simulink model "thermal_analysis"  (R2023b)
settings: Solver=VariableStepAuto  StartTime=0.0  StopTime=1  RelTol=1e-3
values from neighbouring files (symbols this model uses):
  air_temp_init = 75    [run_thermal_analysis.m]
  cap_loss = 194.3    [run_thermal_analysis.m]
  case_temp_init = 75    [run_thermal_analysis.m]
  EMI_loss = 147.1    [run_thermal_analysis.m]
  jyouge_loss = 51.3    [run_thermal_analysis.m]
  module_loss = 426.1    [run_thermal_analysis.m]
  OutTanshi_loss = 94.5    [run_thermal_analysis.m]
  PDC_loss = 16.7    [run_thermal_analysis.m]
  PN_loss = 22.3    [run_thermal_analysis.m]
  PN_temp_init = 82    [run_thermal_analysis.m]
  tanshidai_loss = 514.1    [run_thermal_analysis.m]
libraries: spsSeriesRLCBranchLib x29, spsGroundLib x19, spsControlledCurrentSourceLib x8, spsVoltageMeasurementLib x8, spsACCurrentSourceLib x7, spsDCVoltageSourceLib x3, spsCurrentMeasurementLib x1, sps_lib x1
settings Model: Creator=snow_  LastModifiedBy=snow_
settings DataIOCC: ReturnWorkspaceOutputs=off

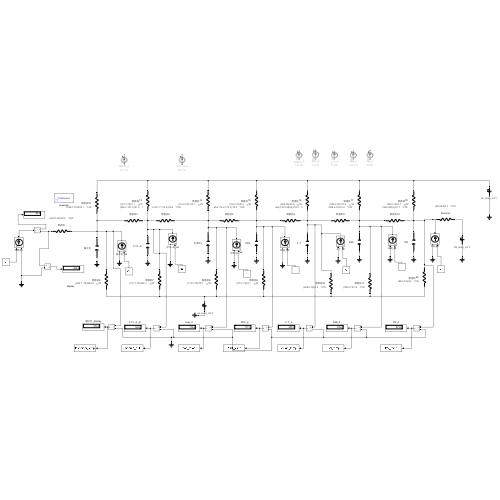
[thumbnail: Simulink's stored preview of the top-level diagram]
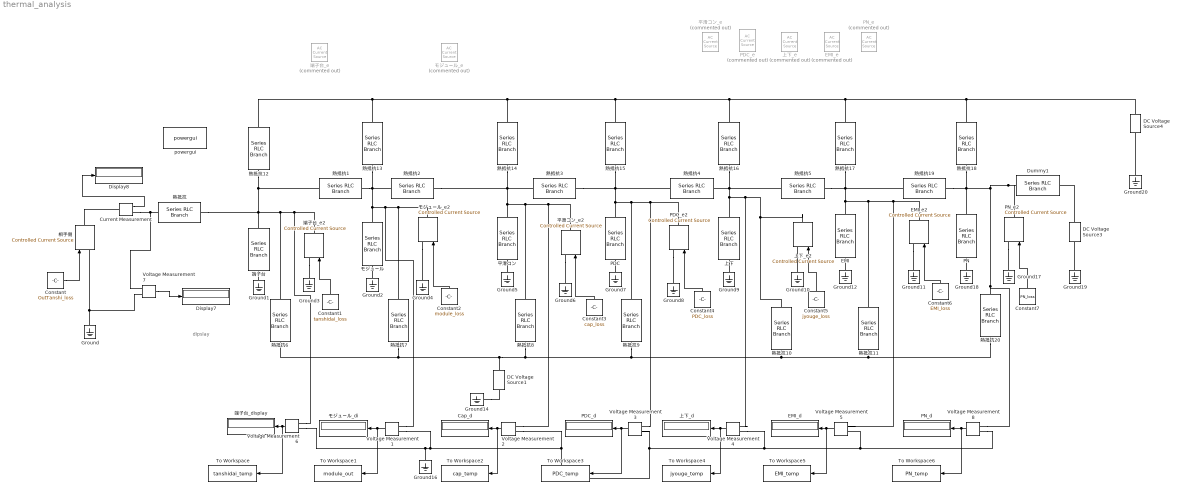
== system thermal_analysis ==
  note: dipslay
  Cap_d : Display
  Constant : Constant  Value=OutTanshi_loss
  Constant1 : Constant  Value=tanshidai_loss
  Constant2 : Constant  Value=module_loss
  Constant3 : Constant  Value=cap_loss
  Constant4 : Constant  Value=PDC_loss
  Constant5 : Constant  Value=jyouge_loss
  Constant6 : Constant  Value=EMI_loss
  Constant7 : Constant  Value=PN_loss
  Current Measurement : spsCurrentMeasurementLib/Current Measurement  PhasorSimulation=off  OutputType=Complex  PSBequivalent=0
  DC Voltage Source1 : spsDCVoltageSourceLib/DC Voltage Source  Amplitude=case_temp_init  Measurements=None
      settings: AttributesFormatString=%<Amplitude>℃
  DC Voltage Source3 : spsDCVoltageSourceLib/DC Voltage Source  Amplitude=PN_temp_init  Measurements=None
      settings: AttributesFormatString=%<Amplitude>℃
  DC Voltage Source4 : spsDCVoltageSourceLib/DC Voltage Source  Amplitude=air_temp_init  Measurements=None
      settings: AttributesFormatString=%<Amplitude>℃
  Display7 : Display
  Display8 : Display
  Dummy1 : spsSeriesRLCBranchLib/Series RLC Branch  LConnTagsString=__new0  RConnTagsString=__new0  BranchType=R  Resistance=(88-82)/50.7  Inductance=1e-3  SetiL0=off  InitialCurrent=0  Capacitance=0.1  Setx0=off  InitialVoltage=0  Measurements=None
      settings: AttributesFormatString=%<Resistance>　℃/W
  EMI : spsSeriesRLCBranchLib/Series RLC Branch  LConnTagsString=__new0  RConnTagsString=__new0  BranchType=C  Resistance=1  Inductance=1e-3  SetiL0=off  InitialCurrent=0  Capacitance=0.1  Setx0=off  InitialVoltage=0  Measurements=None
  EMI_d : Display
  EMI_e : spsACCurrentSourceLib/AC Current Source  Commented=on  Amplitude=147.1  Phase=0  Frequency=0  SampleTime=0  Measurements=None
      settings: AttributesFormatString=%<Amplitude>W  LibrarySourceBlock=sps_lib/Sources/AC Current Source
  EMI_e2 : spsControlledCurrentSourceLib/Controlled Current Source  Initialize=on  Source_Type=AC  Amplitude=0  Phase=0  Frequency=0  Measurements=None
  Ground{,1..12,14,16..20} (19 alike) : spsGroundLib/Ground  LConnTagsString=a
  PDC : spsSeriesRLCBranchLib/Series RLC Branch  LConnTagsString=__new0  RConnTagsString=__new0  BranchType=C  Resistance=1  Inductance=1e-3  SetiL0=off  InitialCurrent=0  Capacitance=0.1  Setx0=off  InitialVoltage=0  Measurements=None
  PDC_d : Display
  PDC_e : spsACCurrentSourceLib/AC Current Source  Commented=on  Amplitude=16.7  Phase=0  Frequency=0  SampleTime=0  Measurements=None
      settings: AttributesFormatString=%<Amplitude>W  LibrarySourceBlock=sps_lib/Sources/AC Current Source
  PDC_e2 : spsControlledCurrentSourceLib/Controlled Current Source  Initialize=on  Source_Type=AC  Amplitude=0  Phase=0  Frequency=0  Measurements=None
  PN : spsSeriesRLCBranchLib/Series RLC Branch  LConnTagsString=__new0  RConnTagsString=__new0  BranchType=C  Resistance=1  Inductance=1e-3  SetiL0=off  InitialCurrent=0  Capacitance=0.1  Setx0=off  InitialVoltage=0  Measurements=None
  PN_d : Display
  PN_e : spsACCurrentSourceLib/AC Current Source  Commented=on  Amplitude=22.3  Phase=0  Frequency=0  SampleTime=0  Measurements=None
      settings: AttributesFormatString=%<Amplitude>W  LibrarySourceBlock=sps_lib/Sources/AC Current Source
  PN_e2 : spsControlledCurrentSourceLib/Controlled Current Source  Initialize=on  Source_Type=AC  Amplitude=0  Phase=0  Frequency=0  Measurements=None
  To Workspace : ToWorkspace  VariableName=tanshidai_temp  SampleTime=-1
  To Workspace1 : ToWorkspace  VariableName=module_out  SampleTime=-1
  To Workspace2 : ToWorkspace  VariableName=cap_temp  SampleTime=-1
  To Workspace3 : ToWorkspace  VariableName=PDC_temp  SampleTime=-1
  To Workspace4 : ToWorkspace  VariableName=jyouge_temp  SampleTime=-1
  To Workspace5 : ToWorkspace  VariableName=EMI_temp  SampleTime=-1
  To Workspace6 : ToWorkspace  VariableName=PN_temp  SampleTime=-1
  Voltage Measurement{1..8} (8 alike) : spsVoltageMeasurementLib/Voltage Measurement  PhasorSimulation=off  OutputType=Complex  PSBequivalent=0
  powergui : sps_lib/powergui  Priority=1  SimulationMode=Continuous  SampleTime=50e-6  frequency=60  Iterations=50  frequencyindice=0  Pbase=100e6  ErrMax=1e-4  UnitsV=kV  UnitsW=MW  buscounter=0  FunctionMessages=off  echomessages=off  EnableUseOfTLC=off  CurrentSourceSwitches=off  DisableSnubberDevices=off  DisableRonSwitches=off  DisableVfSwitches=off  DisplayEquations=off  AutomaticDiscreteSolvers=off  SolverType=Tustin/Backward Euler (TBE)  Interpol=off  ExternalGateDelay=off  methode=off  Ts=100  x0status=blocks  SPID=on  SwTol=0  HookPort=off  NonlinearTolerance=1e-4  nMaxIteration=100  ContinueOnMaxIteration=off  RestoreLinks=warning  ResistiveCurrentMeasurement=off  Frange=[0:2:500]  Ylog=off  Xlog=on  ShowGrid=off  save=off  variable=ZData  structure=0  ZoomFFT=off  StartTime=0.0  cycles=1  DisplayStyle=1  fundamental=60  FreqAxis=off  MaxFrequency=1000  frequencyindicesteady=1  RmsSteady=1  display=off
  モジュール : spsSeriesRLCBranchLib/Series RLC Branch  LConnTagsString=__new0  RConnTagsString=__new0  BranchType=C  Resistance=1  Inductance=1e-3  SetiL0=off  InitialCurrent=0  Capacitance=0.1  Setx0=off  InitialVoltage=0  Measurements=None
  モジュール_di : Display
  モジュール_e : spsACCurrentSourceLib/AC Current Source  Commented=on  Amplitude=426.1  Phase=0  Frequency=0  SampleTime=0  Measurements=None
      settings: AttributesFormatString=%<Amplitude>W  LibrarySourceBlock=sps_lib/Sources/AC Current Source
  モジュール_e2 : spsControlledCurrentSourceLib/Controlled Current Source  Initialize=on  Source_Type=AC  Amplitude=0  Phase=0  Frequency=0  Measurements=None
  上下 : spsSeriesRLCBranchLib/Series RLC Branch  LConnTagsString=__new0  RConnTagsString=__new0  BranchType=C  Resistance=1  Inductance=1e-3  SetiL0=off  InitialCurrent=0  Capacitance=0.1  Setx0=off  InitialVoltage=0  Measurements=None
  上下_d : Display
  上下_e : spsACCurrentSourceLib/AC Current Source  Commented=on  Amplitude=51.3  Phase=0  Frequency=0  SampleTime=0  Measurements=None
      settings: AttributesFormatString=%<Amplitude>W  LibrarySourceBlock=sps_lib/Sources/AC Current Source
  上下_e2 : spsControlledCurrentSourceLib/Controlled Current Source  Initialize=on  Source_Type=AC  Amplitude=0  Phase=0  Frequency=0  Measurements=None
  平滑コン : spsSeriesRLCBranchLib/Series RLC Branch  LConnTagsString=__new0  RConnTagsString=__new0  BranchType=C  Resistance=1  Inductance=1e-3  SetiL0=off  InitialCurrent=0  Capacitance=0.1  Setx0=off  InitialVoltage=0  Measurements=None
  平滑コン_e : spsACCurrentSourceLib/AC Current Source  Commented=on  Amplitude=194.3  Phase=0  Frequency=0  SampleTime=0  Measurements=None
      settings: AttributesFormatString=%<Amplitude>W  LibrarySourceBlock=sps_lib/Sources/AC Current Source
  平滑コン_e2 : spsControlledCurrentSourceLib/Controlled Current Source  Initialize=on  Source_Type=AC  Amplitude=0  Phase=0  Frequency=0  Measurements=None
  熱抵抗 : spsSeriesRLCBranchLib/Series RLC Branch  LConnTagsString=__new0  RConnTagsString=__new0  BranchType=R  Resistance=(269.7-82)/94.5  Inductance=1e-3  SetiL0=off  InitialCurrent=0  Capacitance=0.1  Setx0=off  InitialVoltage=0  Measurements=None
      settings: AttributesFormatString=%<Resistance>　℃/W
  熱抵抗1 : spsSeriesRLCBranchLib/Series RLC Branch  LConnTagsString=__new0  RConnTagsString=__new0  BranchType=R  Resistance=(269.7-101.7)/51.5  Inductance=1e-3  SetiL0=off  InitialCurrent=0  Capacitance=0.1  Setx0=off  InitialVoltage=0  Measurements=None
      settings: AttributesFormatString=%<Resistance>　℃/W
  熱抵抗10 : spsSeriesRLCBranchLib/Series RLC Branch  LConnTagsString=__new0  RConnTagsString=__new0  BranchType=R  Resistance=(289.6-75)/3.5  Inductance=1e-3  SetiL0=off  InitialCurrent=0  Capacitance=0.1  Setx0=off  InitialVoltage=0  Measurements=None
      settings: AttributesFormatString=%<Resistance>　℃/W
  熱抵抗11 : spsSeriesRLCBranchLib/Series RLC Branch  LConnTagsString=__new0  RConnTagsString=__new0  BranchType=R  Resistance=(198.2-75)/12  Inductance=1e-3  SetiL0=off  InitialCurrent=0  Capacitance=0.1  Setx0=off  InitialVoltage=0  Measurements=None
      settings: AttributesFormatString=%<Resistance>　℃/W
  熱抵抗12 : spsSeriesRLCBranchLib/Series RLC Branch  LConnTagsString=__new0  RConnTagsString=__new0  BranchType=R  Resistance=(269.7-75)/260.1  Inductance=1e-3  SetiL0=off  InitialCurrent=0  Capacitance=0.1  Setx0=off  InitialVoltage=0  Measurements=None
      settings: AttributesFormatString=%<Resistance>　℃/W
  熱抵抗13 : spsSeriesRLCBranchLib/Series RLC Branch  LConnTagsString=__new0  RConnTagsString=__new0  BranchType=R  Resistance=(101.7-75)/1.1  Inductance=1e-3  SetiL0=off  InitialCurrent=0  Capacitance=0.1  Setx0=off  InitialVoltage=0  Measurements=None
      settings: AttributesFormatString=%<Resistance>　℃/W
  熱抵抗14 : spsSeriesRLCBranchLib/Series RLC Branch  LConnTagsString=__new0  RConnTagsString=__new0  BranchType=R  Resistance=(174.2-75)/112.1  Inductance=1e-3  SetiL0=off  InitialCurrent=0  Capacitance=0.1  Setx0=off  InitialVoltage=0  Measurements=None
      settings: AttributesFormatString=%<Resistance>　℃/W
  熱抵抗15 : spsSeriesRLCBranchLib/Series RLC Branch  LConnTagsString=__new0  RConnTagsString=__new0  BranchType=R  Resistance=(176.7-75)/8.4  Inductance=1e-3  SetiL0=off  InitialCurrent=0  Capacitance=0.1  Setx0=off  InitialVoltage=0  Measurements=None
      settings: AttributesFormatString=%<Resistance>　℃/W
  熱抵抗16 : spsSeriesRLCBranchLib/Series RLC Branch  LConnTagsString=__new0  RConnTagsString=__new0  BranchType=R  Resistance=(289-75)/20.9  Inductance=1e-3  SetiL0=off  InitialCurrent=0  Capacitance=0.1  Setx0=off  InitialVoltage=0  Measurements=None
      settings: AttributesFormatString=%<Resistance>　℃/W
  熱抵抗17 : spsSeriesRLCBranchLib/Series RLC Branch  LConnTagsString=__new0  RConnTagsString=__new0  BranchType=R  Resistance=(198.2-75)/117.4  Inductance=1e-3  SetiL0=off  InitialCurrent=0  Capacitance=0.1  Setx0=off  InitialVoltage=0  Measurements=None
      settings: AttributesFormatString=%<Resistance>　℃/W
  熱抵抗18 : spsSeriesRLCBranchLib/Series RLC Branch  LConnTagsString=__new0  RConnTagsString=__new0  BranchType=R  Resistance=(88.0-75)/2.7  Inductance=1e-3  SetiL0=off  InitialCurrent=0  Capacitance=0.1  Setx0=off  InitialVoltage=0  Measurements=None
      settings: AttributesFormatString=%<Resistance>　℃/W
  熱抵抗19 : spsSeriesRLCBranchLib/Series RLC Branch  LConnTagsString=__new0  RConnTagsString=__new0  BranchType=R  Resistance=(198.2-88.0)/31.7  Inductance=1e-3  SetiL0=off  InitialCurrent=0  Capacitance=0.1  Setx0=off  InitialVoltage=0  Measurements=None
      settings: AttributesFormatString=%<Resistance>　℃/W
  熱抵抗2 : spsSeriesRLCBranchLib/Series RLC Branch  LConnTagsString=__new0  RConnTagsString=__new0  BranchType=R  Resistance=abs(101.7-174.2)/30.4  Inductance=1e-3  SetiL0=off  InitialCurrent=0  Capacitance=0.1  Setx0=off  InitialVoltage=0  Measurements=None
      settings: AttributesFormatString=%<Resistance>　℃/W
  熱抵抗20 : spsSeriesRLCBranchLib/Series RLC Branch  LConnTagsString=__new0  RConnTagsString=__new0  BranchType=R  Resistance=(88.0-75)/0.6  Inductance=1e-3  SetiL0=off  InitialCurrent=0  Capacitance=0.1  Setx0=off  InitialVoltage=0  Measurements=None
      settings: AttributesFormatString=%<Resistance>　℃/W
  熱抵抗3 : spsSeriesRLCBranchLib/Series RLC Branch  LConnTagsString=__new0  RConnTagsString=__new0  BranchType=R  Resistance=abs(174.2-176.7)/19.0  Inductance=1e-3  SetiL0=off  InitialCurrent=0  Capacitance=0.1  Setx0=off  InitialVoltage=0  Measurements=None
      settings: AttributesFormatString=%<Resistance>　℃/W
  熱抵抗4 : spsSeriesRLCBranchLib/Series RLC Branch  LConnTagsString=__new0  RConnTagsString=__new0  BranchType=R  Resistance=abs(176.5-289.6)/12.9  Inductance=1e-3  SetiL0=off  InitialCurrent=0  Capacitance=0.1  Setx0=off  InitialVoltage=0  Measurements=None
      settings: AttributesFormatString=%<Resistance>　℃/W
  熱抵抗5 : spsSeriesRLCBranchLib/Series RLC Branch  LConnTagsString=__new0  RConnTagsString=__new0  BranchType=R  Resistance=(289.6-75)/14.0  Inductance=1e-3  SetiL0=off  InitialCurrent=0  Capacitance=0.1  Setx0=off  InitialVoltage=0  Measurements=None
      settings: AttributesFormatString=%<Resistance>　℃/W
  熱抵抗6 : spsSeriesRLCBranchLib/Series RLC Branch  LConnTagsString=__new0  RConnTagsString=__new0  BranchType=R  Resistance=(269.7 -75)/294.8  Inductance=1e-3  SetiL0=off  InitialCurrent=0  Capacitance=0.1  Setx0=off  InitialVoltage=0  Measurements=None
      settings: AttributesFormatString=%<Resistance>　℃/W
  熱抵抗7 : spsSeriesRLCBranchLib/Series RLC Branch  LConnTagsString=__new0  RConnTagsString=__new0  BranchType=R  Resistance=(101.7-75)/426.1  Inductance=1e-3  SetiL0=off  InitialCurrent=0  Capacitance=0.1  Setx0=off  InitialVoltage=0  Measurements=None
      settings: AttributesFormatString=%<Resistance>　℃/W
  熱抵抗8 : spsSeriesRLCBranchLib/Series RLC Branch  LConnTagsString=__new0  RConnTagsString=__new0  BranchType=R  Resistance=(174.2-75)/72.7  Inductance=1e-3  SetiL0=off  InitialCurrent=0  Capacitance=0.1  Setx0=off  InitialVoltage=0  Measurements=None
      settings: AttributesFormatString=%<Resistance>　℃/W
  熱抵抗9 : spsSeriesRLCBranchLib/Series RLC Branch  LConnTagsString=__new0  RConnTagsString=__new0  BranchType=R  Resistance=(176.7-75)/2.1  Inductance=1e-3  SetiL0=off  InitialCurrent=0  Capacitance=0.1  Setx0=off  InitialVoltage=0  Measurements=None
      settings: AttributesFormatString=%<Resistance>　℃/W
  相手側 : spsControlledCurrentSourceLib/Controlled Current Source  Initialize=on  Source_Type=AC  Amplitude=0  Phase=0  Frequency=0  Measurements=None
  端子台 : spsSeriesRLCBranchLib/Series RLC Branch  LConnTagsString=__new0  RConnTagsString=__new0  BranchType=C  Resistance=1  Inductance=1e-3  SetiL0=off  InitialCurrent=0  Capacitance=0.1  Setx0=off  InitialVoltage=0  Measurements=None
  端子台_display : Display
  端子台_e : spsACCurrentSourceLib/AC Current Source  Commented=on  Amplitude=514.1  Phase=0  Frequency=0  SampleTime=0  Measurements=None
      settings: AttributesFormatString=%<Amplitude>W  LibrarySourceBlock=sps_lib/Sources/AC Current Source
  端子台_e2 : spsControlledCurrentSourceLib/Controlled Current Source  Initialize=on  Source_Type=AC  Amplitude=0  Phase=0  Frequency=0  Measurements=None
  wires:
  Voltage Measurement1/1 -> To Workspace1/1, モジュール_di/1
  Voltage Measurement3/1 -> To Workspace3/1, PDC_d/1
  Voltage Measurement4/1 -> To Workspace4/1, 上下_d/1
  Voltage Measurement5/1 -> To Workspace5/1, EMI_d/1
  Voltage Measurement6/1 -> To Workspace/1, 端子台_display/1
  Voltage Measurement7/1 -> Display7/1
  Current Measurement/1 -> Display8/1
  Constant/1 -> 相手側/1
  Constant1/1 -> 端子台_e2/1
  Constant2/1 -> モジュール_e2/1
  Constant3/1 -> 平滑コン_e2/1
  Constant4/1 -> PDC_e2/1
  Constant5/1 -> 上下_e2/1
  Constant6/1 -> EMI_e2/1
  Constant7/1 -> PN_e2/1
  Voltage Measurement8/1 -> To Workspace6/1, PN_d/1
  Voltage Measurement2/1 -> To Workspace2/1, Cap_d/1
  connections:
  Ground1/LConn1 -- 端子台/RConn1
  端子台_e2/LConn1 -- Ground3/LConn1
  Ground2/LConn1 -- モジュール/RConn1
  モジュール_e2/LConn1 -- Ground4/LConn1
  平滑コン_e2/LConn1 -- Ground6/LConn1
  Ground5/LConn1 -- 平滑コン/RConn1
  PDC_e2/LConn1 -- Ground8/LConn1
  Ground7/LConn1 -- PDC/RConn1
  上下_e2/LConn1 -- Ground10/LConn1
  Ground9/LConn1 -- 上下/RConn1
  Ground12/LConn1 -- EMI/RConn1
  EMI_e2/LConn1 -- Ground11/LConn1
  熱抵抗/RConn1 -- Voltage Measurement7/LConn1 -- Current Measurement/RConn1
  熱抵抗/LConn1 -- 熱抵抗1/RConn1 -- 熱抵抗12/RConn1 -- 端子台_e2/RConn1 -- Voltage Measurement6/LConn1 -- 熱抵抗6/LConn1 -- 端子台/LConn1
  熱抵抗1/LConn1 -- モジュール_e2/RConn1 -- 熱抵抗7/LConn1 -- Voltage Measurement1/LConn1 -- モジュール/LConn1 -- 熱抵抗13/RConn1 -- 熱抵抗2/RConn1
  熱抵抗2/LConn1 -- 平滑コン_e2/RConn1 -- Voltage Measurement2/LConn1 -- 熱抵抗8/LConn1 -- 平滑コン/LConn1 -- 熱抵抗3/RConn1 -- 熱抵抗14/RConn1
  熱抵抗3/LConn1 -- 熱抵抗4/RConn1 -- PDC_e2/RConn1 -- Voltage Measurement3/LConn1 -- 熱抵抗9/LConn1 -- PDC/LConn1 -- 熱抵抗15/RConn1
  上下/LConn1 -- 上下_e2/RConn1 -- 熱抵抗10/LConn1 -- Voltage Measurement4/LConn1 -- 熱抵抗16/RConn1 -- 熱抵抗5/RConn1 -- 熱抵抗4/LConn1
  熱抵抗5/LConn1 -- 熱抵抗19/RConn1 -- 熱抵抗17/RConn1 -- Voltage Measurement5/LConn1 -- EMI_e2/RConn1 -- 熱抵抗11/LConn1 -- EMI/LConn1
  Ground14/LConn1 -- DC Voltage Source1/LConn1
  DC Voltage Source1/RConn1 -- 熱抵抗6/RConn1 -- 熱抵抗7/RConn1 -- 熱抵抗8/RConn1 -- 熱抵抗10/RConn1 -- 熱抵抗20/RConn1 -- 熱抵抗11/RConn1 -- 熱抵抗9/RConn1
  熱抵抗18/LConn1 -- 熱抵抗16/LConn1 -- 熱抵抗15/LConn1 -- 熱抵抗14/LConn1 -- 熱抵抗13/LConn1 -- 熱抵抗12/LConn1 -- 熱抵抗17/LConn1 -- DC Voltage Source4/RConn1
  Ground16/LConn1 -- Voltage Measurement6/LConn2 -- Voltage Measurement1/LConn2 -- Voltage Measurement2/LConn2 -- Voltage Measurement3/LConn2 -- Voltage Measurement8/LConn2 -- Voltage Measurement5/LConn2 -- Voltage Measurement4/LConn2
  Voltage Measurement8/LConn1 -- 熱抵抗20/LConn1 -- PN_e2/RConn1 -- Dummy1/RConn1 -- 熱抵抗18/RConn1 -- PN/LConn1 -- 熱抵抗19/LConn1
  Ground20/LConn1 -- DC Voltage Source4/LConn1
  Ground19/LConn1 -- DC Voltage Source3/LConn1
  Ground18/LConn1 -- PN/RConn1
  DC Voltage Source3/RConn1 -- Dummy1/LConn1
  PN_e2/LConn1 -- Ground17/LConn1
  Voltage Measurement7/LConn2 -- 相手側/LConn1 -- Ground/LConn1
  相手側/RConn1 -- Current Measurement/LConn1
